simulink model "output_reg_mdl_2021a"  (R2021a)
settings: Solver=VariableStepAuto  StartTime=0.0  StopTime=20  RelTol=1e-3
values from neighbouring files (symbols this model uses):
  ic = 0    [output_reg.m]
  K = acker(A, B, -3 * [1, 1, 1])    [output_reg.m]
  L = acker(transpose(Ae), transpose(Ce),  -2 * [1 , 1, 1, 1, 1])    [output_reg.m]
  omega = 0 *2 * pi    (= 0)    [output_reg.m]
  T = 1e-3    (= 0.001)    [output_reg.m]
  umax = 1    [output_reg.m]
libraries: simulink x2
settings Model: Creator=rapaja  LastModifiedBy=Predrag
settings SolverCC: AlgebraicLoopSolver=TrustRegion
settings RTWCC: DLArmComputeVersion=20.02.1
settings ConfigComp: CovBoundaryAbsTol=1.0e-5

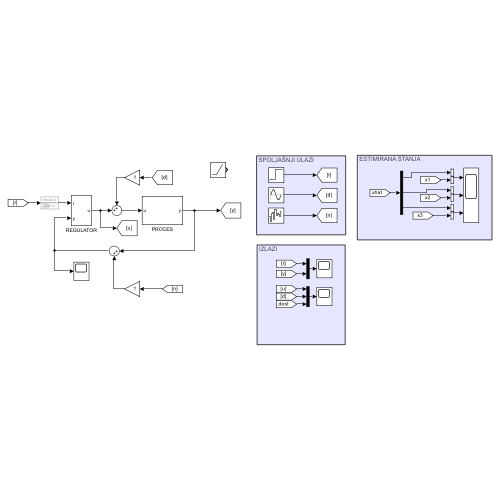
[thumbnail: Simulink's stored preview of the top-level diagram]
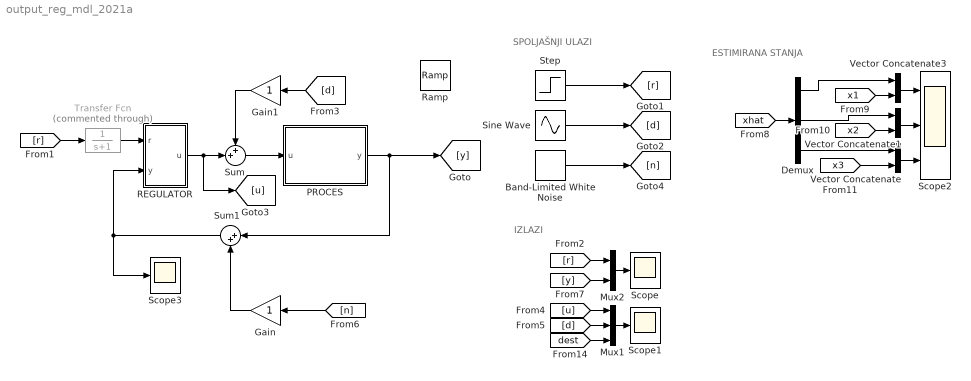
== system output_reg_mdl_2021a ==
  note: ESTIMIRANA STANJA
  note: IZLAZI
  note: SPOLJAŠNJI ULAZI
  Band-Limited White Noise : simulink/Sources/Band-Limited White Noise  Cov=[0.00001]  Ts=T  seed=[23341]
  Demux : Demux  Outputs=3
  Gain : Gain
  Gain1 : Gain
  Mux1 : Mux  Inputs=3
  Mux2 : Mux  Inputs=2
  PROCES : Subsystem
  REGULATOR : Subsystem
  Ramp : simulink/Sources/Ramp  slope=1  start=0  InitialOutput=0
  Scope : Scope
  Scope1 : Scope
  Scope2 : Scope  NumInputPorts=3
  Scope3 : Scope
  Sine Wave : Sin  Frequency=omega  SampleTime=0
  Step : Step  Time=2  SampleTime=0
  Sum : Sum  Inputs=++|
  Sum1 : Sum  Inputs=|++
  Transfer Fcn : TransferFcn  Commented=through  Denominator=[1 1]
  Vector Concatenate : Concatenate
  Vector Concatenate1 : Concatenate
  Vector Concatenate3 : Concatenate
  wires:
  REGULATOR/1(u) -> Sum/2, [u]
  [d] -> Gain1/1
  Band-Limited White Noise/1 -> [n]
  Gain/1 -> Sum1/2
  Gain1/1 -> Sum/1
  [r] -> Mux2/1
  [y] -> Mux2/2
  Mux2/1 -> Scope/1
  Mux1/1 -> Scope1/1
  [u] -> Mux1/1
  [d] -> Mux1/2
  PROCES/1(y) -> Sum1/1, [y]
  Sum/1 -> PROCES/1(u)
  Sum1/1 -> Scope3/1, REGULATOR/2(y)
  Step/1 -> [r]
  [n] -> Gain/1
  [r] -> Transfer Fcn/1
  [xhat] -> Demux/1
  Vector Concatenate/1 -> Scope2/3
  Demux/3 -> Vector Concatenate/1
  [x3] -> Vector Concatenate/2
  Vector Concatenate1/1 -> Scope2/2
  Demux/2 -> Vector Concatenate1/1
  [x2] -> Vector Concatenate1/2
  Vector Concatenate3/1 -> Scope2/1
  [x1] -> Vector Concatenate3/2
  Demux/1 -> Vector Concatenate3/1
  [dest] -> Mux1/3
  Sine Wave/1 -> [d]
  Transfer Fcn/1 -> REGULATOR/1(r)

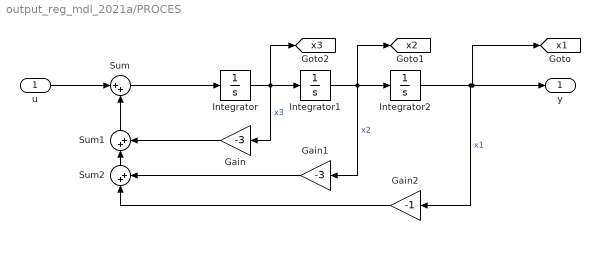
== system output_reg_mdl_2021a/PROCES ==
  u : Inport
  Gain : Gain  Gain=-3
  Gain1 : Gain  Gain=-3
  Gain2 : Gain  Gain=-1
  Integrator : Integrator  InitialCondition=ic
  Integrator1 : Integrator  InitialCondition=ic
  Integrator2 : Integrator  InitialCondition=ic
  Sum : Sum  Inputs=|++
  Sum1 : Sum  Inputs=|++
  Sum2 : Sum  Inputs=|++
  y : Outport
  tag scope: x1=global, x2=global, x3=global
  wires:
  Integrator2/1 -> [x1], y/1, Gain2/1  "x1"
  Integrator1/1 -> [x2], Integrator2/1, Gain1/1  "x2"
  Integrator/1 -> [x3], Integrator1/1, Gain/1  "x3"
  u/1 -> Sum/1
  Sum/1 -> Integrator/1
  Gain/1 -> Sum1/2
  Sum1/1 -> Sum/2
  Sum2/1 -> Sum1/1
  Gain1/1 -> Sum2/2
  Gain2/1 -> Sum2/1

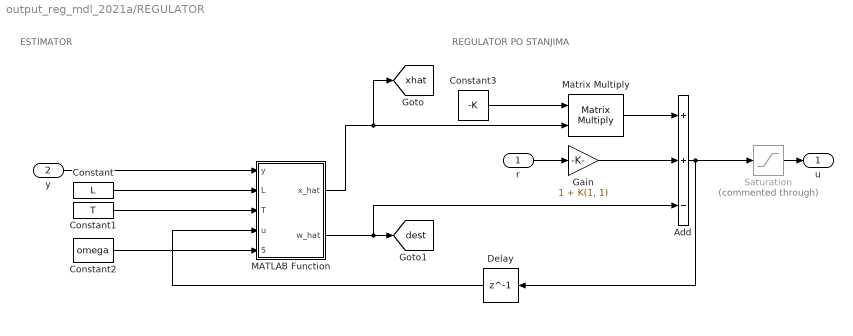
== system output_reg_mdl_2021a/REGULATOR ==
  note: REGULATOR PO STANJIMA
  note: ESTIMATOR
  r : Inport
  y : Inport  Port=2
  Add : Sum  Inputs=++-
  Constant : Constant  Value=L  VectorParams1D=off
  Constant1 : Constant  Value=T
  Constant2 : Constant  Value=omega
  Constant3 : Constant  Value=-K  VectorParams1D=off
  Delay : Delay  DelayLength=1
  Gain : Gain  Gain=1 + K(1, 1)
  MATLAB Function : MATLAB Function  TreatAsAtomicUnit=on
  Matrix Multiply : Product  Multiplication=Matrix(*)
  Saturation : Saturate  Commented=through  UpperLimit=umax  LowerLimit=-umax
  u : Outport
  tag scope: dest=global, xhat=global
  wires:
  y/1 -> MATLAB Function/1(y)
  Constant/1 -> MATLAB Function/2(L)
  Constant1/1 -> MATLAB Function/3(T)
  MATLAB Function/1(x_hat) -> [xhat], Matrix Multiply/2
  MATLAB Function/2(w_hat) -> Add/3, [dest]
  Constant2/1 -> MATLAB Function/5(omega)
  Constant3/1 -> Matrix Multiply/1
  Matrix Multiply/1 -> Add/1
  r/1 -> Gain/1
  Delay/1 -> MATLAB Function/4(u)
  Gain/1 -> Add/2
  Saturation/1 -> u/1
  Add/1 -> Saturation/1, Delay/1

== matlab function output_reg_mdl_2021a/REGULATOR/MATLAB Function ==
  settings: updateMethod=DISCRETE  sampleTime=T
  data: y input; x_hat output; L input; T input; u input; w_hat output; omega input
function [x_hat, w_hat] = fcn(y, L, T, u, omega)
persistent x1hat
persistent x2hat
persistent x3hat
persistent w1hat
persistent w2hat

if(isempty(x1hat))
    x1hat = 0;
end
if(isempty(x2hat))
    x2hat = 0;
end
if(isempty(x3hat))
    x3hat = 0;
end
if(isempty(w1hat))
    w1hat = 0;
end
if(isempty(w2hat))
    w2hat = 0;
end
e = y - x1hat;

x1hat_n = x1hat + T * (x2hat + L(1, 1) * e);
x2hat_n = x2hat + T * (x3hat + L(1, 2) * e);
x3hat_n = x3hat + T * (-3*x3hat - 3*x2hat -x1hat + u + w1hat + L(1, 3) * e);
w1hat_n = w1hat + T * ( w2hat + L(1, 4) * e);
w2hat_n = w2hat + T * (-omega^2 * w1hat +  L(1, 5) * e);

x1hat = x1hat_n;
x2hat = x2hat_n;
x3hat = x3hat_n;
w1hat = w1hat_n;
w2hat = w2hat_n;

x_hat = [x1hat; x2hat; x3hat];
w_hat = w1hat;
